simulink model "Exp2_Observation_2_Delta"  (R2020b)
settings: Solver=VariableStepAuto  StartTime=0.0  StopTime=10.0  RelTol=1e-3
libraries: dsparch4 x1, commutil2 x1, dspsrcs4 x1, dspquant2 x1
settings Model: Creator=Mohit Akhouri  LastModifiedBy=Mohit Akhouri

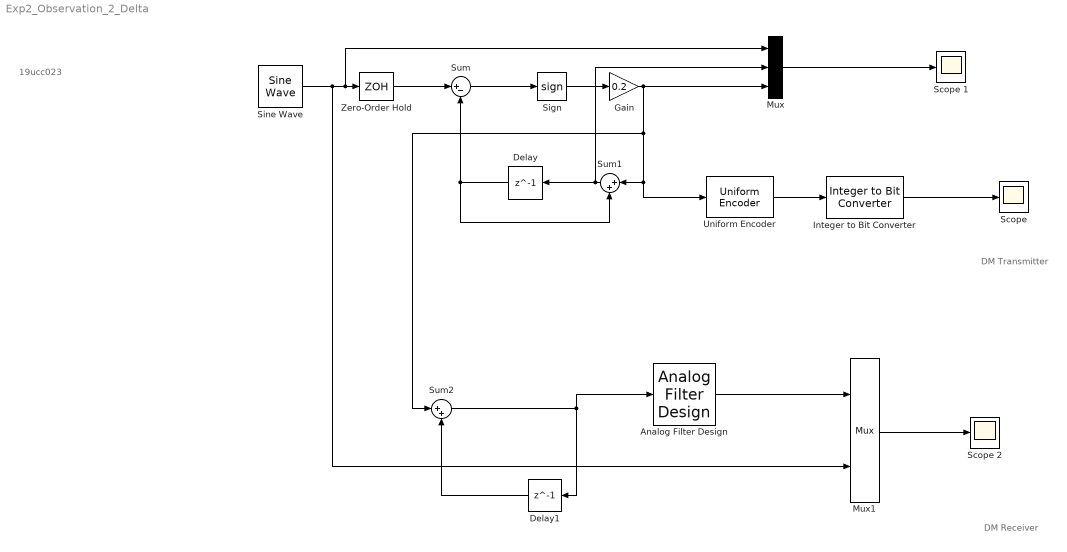
== system Exp2_Observation_2_Delta ==
  note: 19ucc023
  note: DM Receiver
  note: DM Transmitter
  Analog Filter Design : dsparch4/Analog Filter Design  method=Butterworth  filttype=Lowpass  N=8  Wlo=2*pi*1  Whi=80  Rp=2  Rs=40
  Delay : Delay  DelayLength=1
  Delay1 : Delay  DelayLength=1
  Gain : Gain  Gain=0.2
  Integer to Bit Converter : commutil2/Integer to Bit Converter  nbits=2  signedInputValues=Unsigned  bitOrder=MSB first  outDtype=Inherit via internal rule
  Mux : Mux  Inputs=3
  Mux1 : Mux  Inputs=2
  Scope : Scope
  Scope 1 : Scope
  Scope 2 : Scope
  Sign : Signum
  Sine Wave : dspsrcs4/Sine Wave  Amplitude=4  Frequency=1  Phase=0  SampleMode=Discrete  OutComplex=Real  CompMethod=Trigonometric fcn  TableSize=Speed  SampleTime=1/1000  SamplesPerFrame=1  ResetState=Restart at time zero  OutputFrames=off  dataType=double  wordLen=16  udDataType=sfix(16)  fracBitsMode=Best precision  numFracBits=15  OutDataTypeStr=double  LastOutDataTypeStr=double
  Sum : Sum  Inputs=|+-
  Sum1 : Sum  Inputs=|++
  Sum2 : Sum  Inputs=|++
  Uniform Encoder : dspquant2/Uniform Encoder  peak=1  bits=2  otype=Unsigned integer
  Zero-Order Hold : ZeroOrderHold  SampleTime=0.083
  wires:
  Sine Wave/1 -> Mux1/2, Mux/1, Zero-Order Hold/1
  Zero-Order Hold/1 -> Sum/1
  Sum/1 -> Sign/1
  Sign/1 -> Gain/1
  Gain/1 -> Sum2/1, Uniform Encoder/1, Sum1/1, Mux/3
  Mux/1 -> Scope 1/1
  Sum1/1 -> Mux/2, Delay/1
  Delay/1 -> Sum1/2, Sum/2
  Uniform Encoder/1 -> Integer to Bit Converter/1
  Integer to Bit Converter/1 -> Scope/1
  Sum2/1 -> Delay1/1, Analog Filter Design/1
  Delay1/1 -> Sum2/2
  Analog Filter Design/1 -> Mux1/1
  Mux1/1 -> Scope 2/1
